simulink model "LQR_2"  (R2025b)
settings: Solver=VariableStepAuto  StartTime=0.0  StopTime=10.0  RelTol=1e-3
undefined symbols (not defined in the file): ic_xy, ic_xz, ic_yz, K_vert, K_xy, params, rate_lim, T_max
settings Model: Creator=JPham  LastModifiedBy=JPham

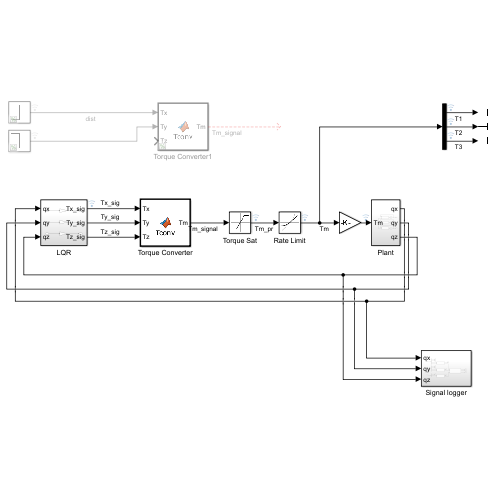
[thumbnail: Simulink's stored preview of the top-level diagram]
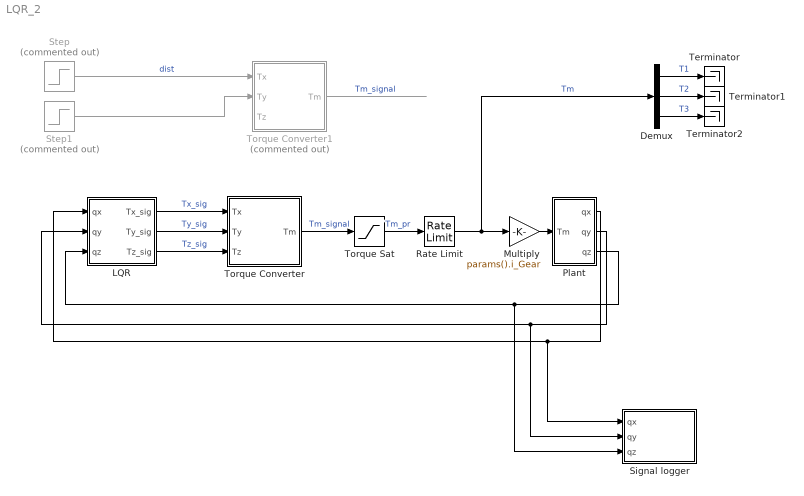
== system LQR_2 ==
  Demux : Demux  Outputs=3
  LQR : Subsystem
  Multiply : Gain  Gain=params().i_Gear
  Plant : Subsystem
  Rate Limit : RateLimiter  RisingSlewLimit=rate_lim  FallingSlewLimit=-rate_lim  SampleTimeMode=inherited
  Signal logger : Subsystem
  Step : Step  Commented=on  Time=2  After=2  SampleTime=0
  Step1 : Step  Commented=on  Time=2  After=-2  SampleTime=0
  Terminator : Terminator
  Terminator1 : Terminator
  Terminator2 : Terminator
  Torque Converter : MATLAB Function  TreatAsAtomicUnit=on
  Torque Converter1 : MATLAB Function  Commented=on  TreatAsAtomicUnit=on
  Torque Sat : Saturate  UpperLimit=T_max  LowerLimit=-T_max
  wires:
  Torque Converter/1(Tm) -> Torque Sat/1  "Tm_signal"
  LQR/1(Tx_sig) -> Torque Converter/1(Tx)  "Tx_sig"
  LQR/2(Ty_sig) -> Torque Converter/2(Ty)  "Ty_sig"
  LQR/3(Tz_sig) -> Torque Converter/3(Tz)  "Tz_sig"
  Plant/2(qy) -> Signal logger/2(qy), LQR/2(qy)
  Plant/1(qx) -> Signal logger/1(qx), LQR/1(qx)
  Plant/3(qz) -> Signal logger/3(qz), LQR/3(qz)
  Demux/1 -> Terminator/1  "T1"
  Demux/2 -> Terminator1/1  "T2"
  Demux/3 -> Terminator2/1  "T3"
  Step/1 -> Torque Converter1/1(Tx)  "dist"
  Step1/1 -> Torque Converter1/2(Ty)
  Multiply/1 -> Plant/1(Tm)
  Torque Converter1/1(Tm) -> ?  "Tm_signal"
  Torque Sat/1 -> Rate Limit/1  "Tm_pr"
  Rate Limit/1 -> Multiply/1, Demux/1  "Tm"

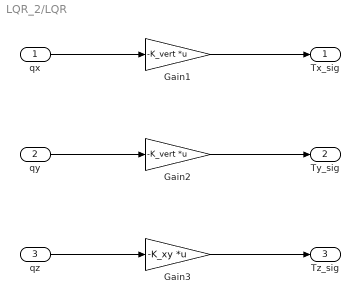
== system LQR_2/LQR ==
  qx : Inport
  qy : Inport  Port=2
  qz : Inport  Port=3
  Gain1 : Gain  Gain=-K_vert  Multiplication=Matrix(K*u) (u vector)
  Gain2 : Gain  Gain=-K_vert  Multiplication=Matrix(K*u) (u vector)
  Gain3 : Gain  Gain=-K_xy  Multiplication=Matrix(K*u) (u vector)
  Tx_sig : Outport
  Ty_sig : Outport  Port=2
  Tz_sig : Outport  Port=3
  wires:
  Gain3/1 -> Tz_sig/1
  qy/1 -> Gain2/1
  Gain1/1 -> Tx_sig/1
  Gain2/1 -> Ty_sig/1
  qz/1 -> Gain3/1
  qx/1 -> Gain1/1

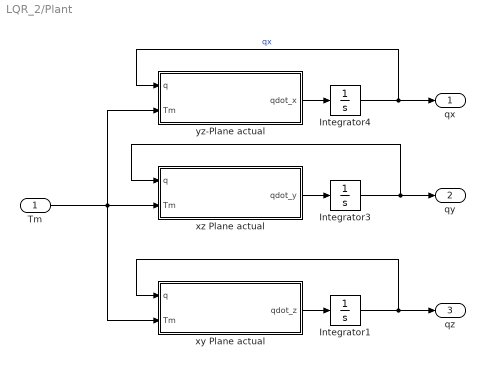
== system LQR_2/Plant ==
  Tm : Inport
  Integrator1 : Integrator  InitialCondition=ic_xy
  Integrator3 : Integrator  InitialCondition=ic_xz  ContinuousStateAttributes='angle'
  Integrator4 : Integrator  InitialCondition=ic_yz  ContinuousStateAttributes='angle'
  xy Plane actual : MATLAB Function  TreatAsAtomicUnit=on
  xz Plane actual : MATLAB Function  TreatAsAtomicUnit=on
  yz-Plane actual : MATLAB Function  TreatAsAtomicUnit=on
  qx : Outport
  qy : Outport  Port=2
  qz : Outport  Port=3
  wires:
  Integrator1/1 -> xy Plane actual/1(q), qz/1
  Tm/1 -> xy Plane actual/2(Tm), yz-Plane actual/2(Tm), xz Plane actual/2(Tm)
  xz Plane actual/1(qdot_y) -> Integrator3/1
  yz-Plane actual/1(qdot_x) -> Integrator4/1
  xy Plane actual/1(qdot_z) -> Integrator1/1
  Integrator4/1 -> yz-Plane actual/1(q), qx/1  "qx"
  Integrator3/1 -> xz Plane actual/1(q), qy/1

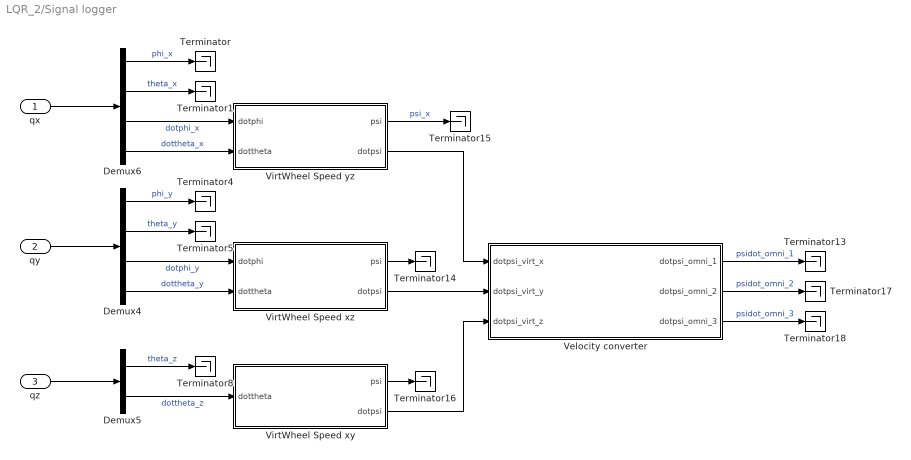
== system LQR_2/Signal logger ==
  qx : Inport
  qy : Inport  Port=2
  qz : Inport  Port=3
  Demux4 : Demux
  Demux5 : Demux  Outputs=2
  Demux6 : Demux
  Terminator{,1,4..5,8,13..18} (11 alike) : Terminator
  Velocity converter : MATLAB Function  TreatAsAtomicUnit=on
  VirtWheel Speed xy : Subsystem
  VirtWheel Speed xz : Subsystem
  VirtWheel Speed yz : Subsystem
  wires:
  Demux4/1 -> Terminator4/1  "phi_y"
  Demux4/4 -> VirtWheel Speed xz/2(dottheta)  "dottheta_y"
  Demux6/4 -> VirtWheel Speed yz/2(dottheta)  "dottheta_x"
  Demux6/1 -> Terminator/1  "phi_x"
  Demux4/2 -> Terminator5/1  "theta_y"
  Demux6/3 -> VirtWheel Speed yz/1(dotphi)  "dotphi_x"
  Demux6/2 -> Terminator1/1  "theta_x"
  Demux5/2 -> VirtWheel Speed xy/1(dottheta)  "dottheta_z"
  Demux5/1 -> Terminator8/1  "theta_z"
  Demux4/3 -> VirtWheel Speed xz/1(dotphi)  "dotphi_y"
  VirtWheel Speed yz/1(psi) -> Terminator15/1  "psi_x"
  VirtWheel Speed xy/2(dotpsi) -> Velocity converter/3(dotpsi_virt_z)
  VirtWheel Speed xy/1(psi) -> Terminator16/1
  VirtWheel Speed yz/2(dotpsi) -> Velocity converter/1(dotpsi_virt_x)
  VirtWheel Speed xz/2(dotpsi) -> Velocity converter/2(dotpsi_virt_y)
  VirtWheel Speed xz/1(psi) -> Terminator14/1
  Velocity converter/1(dotpsi_omni_1) -> Terminator13/1  "psidot_omni_1"
  Velocity converter/3(dotpsi_omni_3) -> Terminator18/1  "psidot_omni_3"
  Velocity converter/2(dotpsi_omni_2) -> Terminator17/1  "psidot_omni_2"
  qy/1 -> Demux4/1
  qx/1 -> Demux6/1
  qz/1 -> Demux5/1

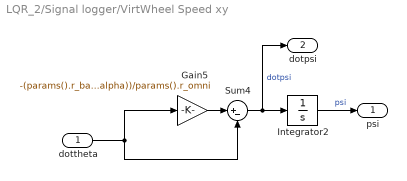
== system LQR_2/Signal logger/VirtWheel Speed xy ==
  dottheta : Inport
  Gain5 : Gain  Gain=-(params().r_ball*sin(params().alpha))/params().r_omni
  Integrator2 : Integrator
  Sum4 : Sum  Inputs=|+-
  psi : Outport
  dotpsi : Outport  Port=2
  wires:
  Integrator2/1 -> psi/1  "psi"
  Sum4/1 -> Integrator2/1, dotpsi/1  "dotpsi"
  dottheta/1 -> Sum4/2, Gain5/1
  Gain5/1 -> Sum4/1

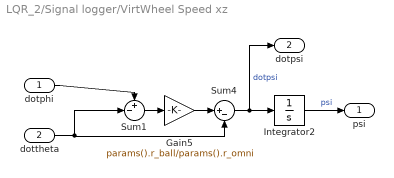
== system LQR_2/Signal logger/VirtWheel Speed xz ==
  dotphi : Inport
  dottheta : Inport  Port=2
  Gain5 : Gain  Gain=params().r_ball/params().r_omni
  Integrator2 : Integrator
  Sum1 : Sum  Inputs=+-|
  Sum4 : Sum  Inputs=|+-
  psi : Outport
  dotpsi : Outport  Port=2
  wires:
  Gain5/1 -> Sum4/1
  dottheta/1 -> Sum1/2, Sum4/2
  Sum4/1 -> dotpsi/1, Integrator2/1  "dotpsi"
  Integrator2/1 -> psi/1  "psi"
  dotphi/1 -> Sum1/1
  Sum1/1 -> Gain5/1

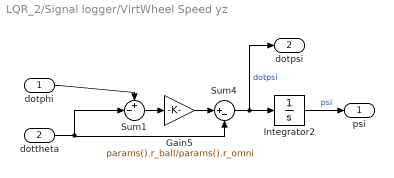
== system LQR_2/Signal logger/VirtWheel Speed yz ==
  dotphi : Inport
  dottheta : Inport  Port=2
  Gain5 : Gain  Gain=params().r_ball/params().r_omni
  Integrator2 : Integrator
  Sum1 : Sum  Inputs=+-|
  Sum4 : Sum  Inputs=|+-
  psi : Outport
  dotpsi : Outport  Port=2
  wires:
  Sum1/1 -> Gain5/1
  dotphi/1 -> Sum1/1
  Integrator2/1 -> psi/1  "psi"
  Sum4/1 -> Integrator2/1, dotpsi/1  "dotpsi"
  dottheta/1 -> Sum4/2, Sum1/2
  Gain5/1 -> Sum4/1

== matlab function LQR_2/Signal logger/Velocity converter ==
  data: dotpsi_virt_x input; dotpsi_virt_y input; dotpsi_omni_1 output; dotpsi_virt_z input; dotpsi_omni_2 output; dotpsi_omni_3 output
% This function convert the velocity of the virtual wheels
% from three planes to the velocity of the omniwheels.
% for beta = 0

function [dotpsi_omni_1, dotpsi_omni_2, dotpsi_omni_3] = ...
    omni_velocity_from_virt(dotpsi_virt_x, dotpsi_virt_y, dotpsi_virt_z)
bb = params();
rads_to_rpm = 30/pi;

dotpsi_omni_1 = (dotpsi_virt_x * cos(bb.alpha) ...
    + dotpsi_virt_z*sin(bb.alpha))*rads_to_rpm;
dotpsi_omni_2 = (-0.5 * dotpsi_virt_x * cos(bb.alpha) ...
    - sqrt(3)*dotpsi_virt_y*cos(bb.alpha)/2 ...
    + dotpsi_virt_z*sin(bb.alpha))* rads_to_rpm;
dotpsi_omni_3 = (-0.5 * dotpsi_virt_x * cos(bb.alpha) ...
    + sqrt(3)*dotpsi_virt_y*cos(bb.alpha)/2 ...
    + dotpsi_virt_z*sin(bb.alpha))* rads_to_rpm;
end

== matlab function LQR_2/Torque Converter1 ==
  data: Tx input; Ty input; Tm output; Tz input
function Tm = Tconv(Tx, Ty, Tz)
    alpha = params().alpha;
    beta  = params().beta;
    % Omni to motors torque convert matrix
    T_o2m = (1/(3*cos(alpha)))*...
    [2*cos(beta)                  , -2*sin(beta)                , cos(alpha);
    (-sqrt(3)*sin(beta)-cos(beta)), (sin(beta)-sqrt(3)*cos(beta)), cos(alpha);
     (sqrt(3)*sin(beta)-cos(beta)), (sin(beta)+sqrt(3)*cos(beta)), cos(alpha)
    ];
    Tm = T_o2m*[Tx; Ty; Tz];
    Tm = Tm./params().i_Gear;
end

== matlab function LQR_2/Torque Converter ==
  data: Tx input; Ty input; Tm output; Tz input
function Tm = Tconv(Tx, Ty, Tz)
    alpha = params().alpha;
    beta  = params().beta;
    % Omni to motors torque convert matrix
    T_o2m = (1/(3*cos(alpha)))*...
    [2*cos(beta)                  , -2*sin(beta)                , cos(alpha);
    (-sqrt(3)*sin(beta)-cos(beta)), (sin(beta)-sqrt(3)*cos(beta)), cos(alpha);
     (sqrt(3)*sin(beta)-cos(beta)), (sin(beta)+sqrt(3)*cos(beta)), cos(alpha)
    ];
    Tm = T_o2m*[Tx; Ty; Tz];
    Tm = Tm./params().i_Gear;
end

== matlab function LQR_2/Plant/xy Plane actual ==
  data: q input; Tm input; qdot_z output
function qdot_z = f(q, Tm)
    % Define dimensions for code generation
    % x is 2x1 state: [theta; theta_dot]
    % Tm is the torques from 3 motors
    % p is the parameter structure
    
    theta   = q(1); % theta
    dottheta= q(2); % theta_dot
    alpha = params().alpha;
    beta  = params().beta;
    Tz = Tm(1) + Tm(2) + Tm(3);

    p = params;
    
    T_f = ((p.r_ball*p.r_omni*p.Theta_body_xy*sin(p.alpha))...
        /((p.r_omni)^2*p.Theta_body_xy+(p.r_ball)^2*p.Theta_virt_xy*(sin(p.alpha))^2))*Tz;

    ddottheta = -(p.r_ball*sin(p.alpha))*(p.r_ball*p.Theta_virt_xy*sin(p.alpha)+p.r_omni*p.Theta_ball)*T_f...
        /((p.r_omni)^2*p.Theta_body_xy*p.Theta_ball+(p.r_ball)^2*(p.Theta_body_xy+p.Theta_ball)*p.Theta_virt_xy*(sin(p.alpha))^2);
    
    % Assemble qdot_z
    qdot_z = [dottheta;
                ddottheta];
end

== matlab function LQR_2/Plant/xz Plane actual ==
  data: q input; Tm input; qdot_y output
function qdot_y = f(q, Tm)
    % Define dimensions for code generation
    % x is 4x1 state: [phi; theta; phi_dot; theta_dot]
    % Tm is the torque from the three motors
    % p is the parameter structure

    % Convert motor torque to omniwheel torque
    alpha = params().alpha;
    beta  = params().beta;
    Ty = cos(alpha)*(-Tm(1)*sin(beta)) - Tm(2)*cos(beta + pi/6) + Tm(3)*cos(beta - pi/6);

    % States
    phi     = q(1); % phi
    theta   = q(2); % theta
    dotphi  = q(3); % phi_dot
    dottheta= q(4); % theta_dot
    
    p = params;
    % Aux Parameters
    m_tot = p.m_ball + p.m_body + p.m_virt;
    r_tot = p.r_ball + p.r_omni;
    gamma = p.l*p.m_body + (p.r_ball + p.r_omni)*p.m_virt;
    
    % M matrix
    M11 = m_tot * p.r_ball^2 + p.Theta_ball + (p.r_ball / p.r_omni)^2 * p.Theta_virt_vertical;
    M12 = -(p.r_ball / p.r_omni^2) * r_tot * p.Theta_virt_vertical + gamma * p.r_ball*cos(theta); 
    M22 = (r_tot^2 / p.r_omni^2) * p.Theta_virt_vertical + p.Theta_body_vertical + ...
           p.m_body * p.l^2 + p.m_virt * r_tot^2;
    M21 = M12;

    M = [M11, M12;
         M21, M22];
    
    % C vector
    Cvec = [ -p.r_ball*gamma*sin(theta)*dottheta^2; 
              0 ];
    % G vector
    Gvec = [ 0; 
            -p.g*sin(theta)*gamma ];
    % S vector (f_NP = S*u(t))
    S = [ p.r_ball / p.r_omni; -p.r_ball / p.r_omni ];
    
    % --- Dynamics Calculation ---
    F_np = S * Ty; 
    
    % Solve for qdd from M * qdd + C + G = F_np
    % qddot = M \ (F_np - C - G) = [theta_doubledot; phi_doubledot]
    qddot = M \ (F_np - Cvec - Gvec);
    
    % Assemble qdot_y
    qdot_y = [dotphi;
              dottheta;
              qddot(1);
              qddot(2)];
end

== matlab function LQR_2/Plant/yz-Plane actual ==
  data: q input; Tm input; qdot_x output
function qdot_x = f(q, Tm)
    % Define dimensions for code generation
    % x is 4x1 state: [phi; theta; phi_dot; theta_dot]
    % Tm is the torque from the three motors
    % p is the parameter structure, loaded into simulink in Model Explorer

    % Convert motor torque to omniwheel torque
    alpha = params().alpha;
    beta  = params().beta;
    Tx = cos(alpha)*(Tm(1)*cos(beta)) - Tm(2)*sin(beta + pi/6) + Tm(3)*sin(beta - pi/6);

    % States
    phi     = q(1); % phi
    theta   = q(2); % theta
    dotphi  = q(3); % phi_dot
    dottheta= q(4); % theta_dot
    
    p = params;
    % Aux Parameters
    m_tot = p.m_ball + p.m_body + p.m_virt;
    r_tot = p.r_ball + p.r_omni;
    gamma = p.l*p.m_body + (p.r_ball + p.r_omni)*p.m_virt;
    
    % M matrix
    M11 = m_tot * p.r_ball^2 + p.Theta_ball + (p.r_ball / p.r_omni)^2 * p.Theta_virt_vertical;
    M12 = -(p.r_ball / p.r_omni^2) * r_tot * p.Theta_virt_vertical + gamma * p.r_ball*cos(theta); 
    M22 = (r_tot^2 / p.r_omni^2) * p.Theta_virt_vertical + p.Theta_body_vertical + ...
           p.m_body * p.l^2 + p.m_virt * r_tot^2;
    M21 = M12;

    M = [M11, M12;
         M21, M22];
    
    % C vector
    Cvec = [ -p.r_ball*gamma*sin(theta)*dottheta^2; 
              0 ];
    % G vector
    Gvec = [ 0; 
            -p.g*sin(theta)*gamma ];
    % S vector (f_NP = S*u(t))
    S = [ p.r_ball / p.r_omni; -p.r_ball / p.r_omni ];
    
    % --- Dynamics Calculation ---
    F_np = S * Tx; 
    
    % Solve for qdd from M * qdd + C + G = F_np
    % qddot = M \ (F_np - C - G) = [theta_doubledot; phi_doubledot]
    qddot = M \ (F_np - Cvec - Gvec);
    
    % Assemble qdot_vertical
    qdot_x = [dotphi;
              dottheta;
              qddot(1);
              qddot(2)];
end
